simulink model "nonlinear_model"  (R2016a)
settings: Solver=VariableStepAuto  StartTime=0.0  StopTime=T  MaxStep=1e-3  RelTol=1e-3
values from neighbouring files (symbols this model uses):
  a = 0.025    [constants.m]
  A = [ 0     0     0     0     1     0     0     0 ... (first row only)    [reduced_state_space.m]
  angular_velocity_0 = [0 0 0]    [simulation.m]
  B = [0 0 0 0 b_11 0    0    b_51 ... (first row only)    [reduced_state_space.m]
  C = [c_11 0    0    c_15 0 0 0 0 ... (first row only)    [reduced_state_space.m]
  g = 9.81305    [constants.m]
  h = 0.0095    [constants.m]
  I = [I_1  0    0 ... (first row only)    [constants.m]
  K = lqr(A, B, Q, R)    [reduced_state_space.m]
  Kr = (lqr(A',C',Q_r,R_r))'    [reduced_state_space.m]
  Ks = pocet_zavitu * prumerna_area    (= 0.0603185789489)    [constants.m]
  m = pi*r^2*h*neodymium_density    (= 0.0694645405617)    [constants.m]
  m_0 = 3.3906    [constants.m]
  m_2 = 1.5321    [constants.m]
  max_I = 2    [constants.m]
  noise_power = 1*10^(-11)    (= 1e-11)    [constants.m]
  perm_vak_4pi = 10^(-7)    (= 1e-07)    [constants.m]
  phi_0 = [0.00 0.00 0]    [simulation.m]
  R = [1 0 ... (first row only)    [reduced_state_space.m]
  rot_damp = 0*0.00002    (= 0)    [constants.m]
  s = 1*0.001    (= 0.001)    [constants.m]
  sample_period = 0.003    [constants.m]
  setpoint_x = perm_vak_4pi*m_0 * ( (3*s*z_r)/(s^2+z_r^2)^(5/2) )    [simulation.m]
  setpoint_y = setpoint_x    [simulation.m]
  x_0 = [0.001 -0.0015 z_r-0.000]    [simulation.m]
  x_1 = [-a  a 0]    [constants.m]
  x_2 = [ a  a 0]    [constants.m]
  x_3 = [-a -a 0]    [constants.m]
  x_4 = [ a -a 0]    [constants.m]
  x_5 = [ 0  a 0]    [constants.m]
  x_6 = [-a  0 0]    [constants.m]
  x_7 = [ a  0 0]    [constants.m]
  x_8 = [ 0 -a 0]    [constants.m]
undefined symbols (not defined in the file or in its folder): Kd, Ki, Kp, X, Y, Z
libraries: sm_lib x27, nesl_utility x9, simulink x8, vrlib x1
(part 2 of 2)

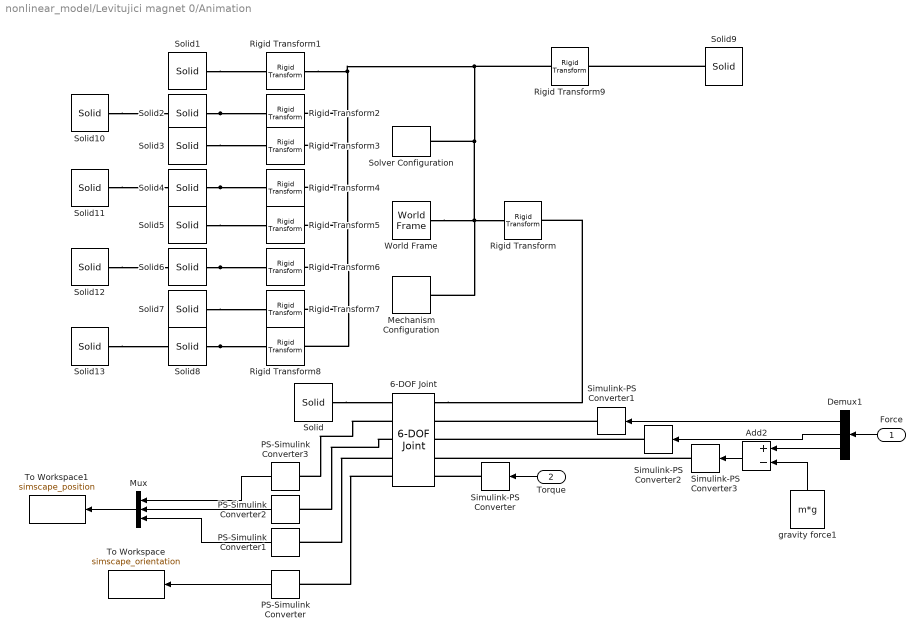
== system nonlinear_model/Levitujici magnet 0/Animation ==
  Force : Inport
  Torque : Inport  Port=2
  6-DOF Joint : sm_lib/Joints/6-DOF Joint  SenseConstraintForce=off  SenseConstraintForceX=off  SenseConstraintForceY=off  SenseConstraintForceZ=off  SenseConstraintTorque=off  SenseConstraintTorqueX=off  SenseConstraintTorqueY=off  SenseConstraintTorqueZ=off  SenseTotalForce=off  SenseTotalForceX=off  SenseTotalForceY=off  SenseTotalForceZ=off  SenseTotalTorque=off  SenseTotalTorqueX=off  SenseTotalTorqueY=off  SenseTotalTorqueZ=off  CompositeWrenchDir=FollowerOnBase  CompositeWrenchFrame=BaseFrame  PxEquilibriumPosition=0  PxEquilibriumPositionUnits=m  PxSpringStiffness=0  PxSpringStiffnessUnits=N/m  PxDampingCoefficient=0  PxDampingCoefficientUnits=N/(m/s)  PxTorqueActuationMode=InputTorque  PxMotionActuationMode=ComputedMotion  PxSensePosition=on  PxSenseVelocity=off  PxSenseAcceleration=off  PxSenseTorqueForce=off  PxPositionTargetSpecify=on  PxPositionTargetPriority=High  PxPositionTargetValue=x_0(1)  PxPositionTargetValueUnits=m  PxVelocityTargetSpecify=off  PxVelocityTargetPriority=High  PxVelocityTargetValue=0  PxVelocityTargetValueUnits=m/s  PyEquilibriumPosition=0  PyEquilibriumPositionUnits=m  PySpringStiffness=0  PySpringStiffnessUnits=N/m  PyDampingCoefficient=0  PyDampingCoefficientUnits=N/(m/s)  PyTorqueActuationMode=InputTorque  PyMotionActuationMode=ComputedMotion  PySensePosition=on  PySenseVelocity=off  PySenseAcceleration=off  PySenseTorqueForce=off  PyPositionTargetSpecify=on  PyPositionTargetPriority=High  PyPositionTargetValue=x_0(2)  PyPositionTargetValueUnits=m  PyVelocityTargetSpecify=off  PyVelocityTargetPriority=High  PyVelocityTargetValue=0  PyVelocityTargetValueUnits=m/s  PzEquilibriumPosition=0  PzEquilibriumPositionUnits=m  PzSpringStiffness=0  PzSpringStiffnessUnits=N/m  PzDampingCoefficient=0  PzDampingCoefficientUnits=N/(m/s)  PzTorqueActuationMode=InputTorque  PzMotionActuationMode=ComputedMotion  PzSensePosition=on  PzSenseVelocity=off  PzSenseAcceleration=off  PzSenseTorqueForce=off  PzPositionTargetSpecify=on  PzPositionTargetPriority=High  PzPositionTargetValue=x_0(3)  PzPositionTargetValueUnits=m  PzVelocityTargetSpecify=off  PzVelocityTargetPriority=High  PzVelocityTargetValue=0  PzVelocityTargetValueUnits=m/s  SphDefPosRotationMethod=None  SphDefPosRotationAngleUnits=deg  SphDefPosRotationStandardAxis=+Z  SphDefPosRotationAngle=0.0  SphDefPosRotationArbitraryAxis=[0 0 1]  SphDefPosFollAlignAxisA=+X  SphDefPosBaseAlignAxisA=+Y  SphDefPosFollAlignAxisB=+Y  SphDefPosBaseAlignAxisB=+Z  SphDefPosRotationSequenceAxes=FollowerAxes  SphDefPosRotationSequence=XYX  SphDefPosRotationSequenceAngles=[0 0 0]  SphDefPosRotationSequenceAnglesUnits=deg  SphDefPosRotationMatrix=[1 0 0; 0 1 0; 0 0 1]  SphEqPosRotationMethod=None  SphEqPosRotationAngleUnits=deg  SphEqPosRotationStandardAxis=+Z  SphEqPosRotationAngle=0.0  SphEqPosRotationArbitraryAxis=[0 0 1]  SphEqPosFollAlignAxisA=+X  SphEqPosBaseAlignAxisA=+Y  SphEqPosFollAlignAxisB=+Y  SphEqPosBaseAlignAxisB=+Z  SphEqPosRotationSequenceAxes=FollowerAxes  SphEqPosRotationSequence=XYX  SphEqPosRotationSequenceAngles=[0 0 0]  SphEqPosRotationSequenceAnglesUnits=deg  SphEqPosRotationMatrix=[1 0 0; 0 1 0; 0 0 1]  SphSpringStiffness=0  SphSpringStiffnessUnits=N*m/deg  SphDampingCoefficient=rot_damp_sim  SphDampingCoefficientUnits=N*m/(deg/s)  SphActuateTorqueX=off  SphActuateTorqueY=off  SphActuateTorqueZ=off  SphActuateTorque=on  SphTorqueActuationMode=InputTorque  SphMotionActuationMode=ComputedMotion  SphActuationFrame=BaseFrame  SphSensePosition=on  SphSenseVelocityX=off  SphSenseVelocityY=off  SphSenseVelocityZ=off  SphSenseVelocity=off  SphSenseAccelerationX=off  SphSenseAccelerationY=off  SphSenseAccelerationZ=off  SphSenseAcceleration=off  SphSenseTorqueX=off  SphSenseTorqueY=off  SphSenseTorqueZ=off  SphSenseTorqueForce=off  SphSensingFrame=BaseFrame  SphPositionTargetRotationMethod=RotationSequence  SphPositionTargetRotationAngleUnits=deg  SphPositionTargetRotationStandardAxis=+Z  SphPositionTargetRotationAngle=0.0  SphPositionTargetRotationArbitraryAxis=[0 0 1]  SphPositionTargetFollAlignAxisA=+X  SphPositionTargetBaseAlignAxisA=+Y  SphPositionTargetFollAlignAxisB=+Y  SphPositionTargetBaseAlignAxisB=+Z  SphPositionTargetRotationSequenceAxes=FollowerAxes  SphPositionTargetRotationSequence=ZYX  SphPositionTargetRotationSequenceAngles=[phi_0(3), phi_0(2), phi_0(1)]  SphPositionTargetRotationSequenceAnglesUnits=rad  SphPositionTargetRotationMatrix=[1 0 0; 0 1 0; 0 0 1]  SphPositionTargetSpecify=on  SphPositionTargetPriority=High  SphVelocityTargetValue=[angular_velocity_0(3), angular_velocity_0(2), angular_velocity_0(1)]  SphVelocityTargetValueUnits=deg/s  SphVelocityTargetSpecify=on  SphVelocityTargetPriority=High  SphVelocityTargetInFollowerFrame=on
  Add2 : Sum  Inputs=+-
  Demux1 : Demux  Outputs=3
  Mechanism Configuration : sm_lib/Utilities/Mechanism Configuration  UniformGravity=Constant  GravityVector=[0 0 -0]  GravityUnits=m/s^2  LinearizationDelta=0.001
  Mux : Mux  Inputs=3
  PS-Simulink Converter{,1..3} (4 alike) : nesl_utility/PS-Simulink Converter  PhysicalDomain=network_engine_domain  SubClassName=ps_output  LeftPortType=input  RightPortType=output  PseudoPeriodic=off  Frequencies=[]  Unit=1  AffineConversion=off
  Rigid Transform : sm_lib/Frames and Transforms/Rigid Transform  TranslationMethod=None  TranslationLengthUnit=m  TranslationStandardAxis=+Z  TranslationStandardOffset=0  TranslationCartesianOffset=[]  TranslationROffset=0  TranslationROffsetUnits=m  TranslationZOffset=0  TranslationZOffsetUnits=m  TranslationThetaOffset=0  TranslationThetaOffsetUnits=deg  RotationMethod=None  RotationAngleUnits=deg  RotationStandardAxis=+Z  RotationAngle=0.0  RotationArbitraryAxis=[0 0 1]  FollAlignAxisA=+X  BaseAlignAxisA=+Y  FollAlignAxisB=+Y  BaseAlignAxisB=+Z  RotationSequenceAxes=FollowerAxes  RotationSequence=ZXY  RotationSequenceAngles=[phi_0(3), phi_0(2), phi_0(1)]  RotationSequenceAnglesUnits=rad  RotationMatrix=[1 0 0; 0 1 0; 0 0 1]
  Rigid Transform1 : sm_lib/Frames and Transforms/Rigid Transform  TranslationMethod=Cartesian  TranslationLengthUnit=m  TranslationStandardAxis=+Z  TranslationStandardOffset=0  TranslationCartesianOffset=x_1-[0 0 0.0055]  TranslationROffset=0  TranslationROffsetUnits=m  TranslationZOffset=0  TranslationZOffsetUnits=m  TranslationThetaOffset=0  TranslationThetaOffsetUnits=deg  RotationMethod=None  RotationAngleUnits=deg  RotationStandardAxis=+Z  RotationAngle=0.0  RotationArbitraryAxis=[0 0 1]  FollAlignAxisA=+X  BaseAlignAxisA=+Y  FollAlignAxisB=+Y  BaseAlignAxisB=+Z  RotationSequenceAxes=FollowerAxes  RotationSequence=XYX  RotationSequenceAngles=[0 0 0]  RotationSequenceAnglesUnits=deg  RotationMatrix=[1 0 0; 0 1 0; 0 0 1]
  Rigid Transform2 : sm_lib/Frames and Transforms/Rigid Transform  TranslationMethod=Cartesian  TranslationLengthUnit=m  TranslationStandardAxis=+Z  TranslationStandardOffset=0  TranslationCartesianOffset=x_5-[0 0 0.0055]  TranslationROffset=0  TranslationROffsetUnits=m  TranslationZOffset=0  TranslationZOffsetUnits=m  TranslationThetaOffset=0  TranslationThetaOffsetUnits=deg  RotationMethod=None  RotationAngleUnits=deg  RotationStandardAxis=+Z  RotationAngle=0.0  RotationArbitraryAxis=[0 0 1]  FollAlignAxisA=+X  BaseAlignAxisA=+Y  FollAlignAxisB=+Y  BaseAlignAxisB=+Z  RotationSequenceAxes=FollowerAxes  RotationSequence=XYX  RotationSequenceAngles=[0 0 0]  RotationSequenceAnglesUnits=deg  RotationMatrix=[1 0 0; 0 1 0; 0 0 1]
  Rigid Transform3 : sm_lib/Frames and Transforms/Rigid Transform  TranslationMethod=Cartesian  TranslationLengthUnit=m  TranslationStandardAxis=+Z  TranslationStandardOffset=0  TranslationCartesianOffset=x_2-[0 0 0.0055]  TranslationROffset=0  TranslationROffsetUnits=m  TranslationZOffset=0  TranslationZOffsetUnits=m  TranslationThetaOffset=0  TranslationThetaOffsetUnits=deg  RotationMethod=None  RotationAngleUnits=deg  RotationStandardAxis=+Z  RotationAngle=0.0  RotationArbitraryAxis=[0 0 1]  FollAlignAxisA=+X  BaseAlignAxisA=+Y  FollAlignAxisB=+Y  BaseAlignAxisB=+Z  RotationSequenceAxes=FollowerAxes  RotationSequence=XYX  RotationSequenceAngles=[0 0 0]  RotationSequenceAnglesUnits=deg  RotationMatrix=[1 0 0; 0 1 0; 0 0 1]
  Rigid Transform4 : sm_lib/Frames and Transforms/Rigid Transform  TranslationMethod=Cartesian  TranslationLengthUnit=m  TranslationStandardAxis=+Z  TranslationStandardOffset=0  TranslationCartesianOffset=x_6-[0 0 0.0055]  TranslationROffset=0  TranslationROffsetUnits=m  TranslationZOffset=0  TranslationZOffsetUnits=m  TranslationThetaOffset=0  TranslationThetaOffsetUnits=deg  RotationMethod=None  RotationAngleUnits=deg  RotationStandardAxis=+Z  RotationAngle=0.0  RotationArbitraryAxis=[0 0 1]  FollAlignAxisA=+X  BaseAlignAxisA=+Y  FollAlignAxisB=+Y  BaseAlignAxisB=+Z  RotationSequenceAxes=FollowerAxes  RotationSequence=XYX  RotationSequenceAngles=[0 0 0]  RotationSequenceAnglesUnits=deg  RotationMatrix=[1 0 0; 0 1 0; 0 0 1]
  Rigid Transform5 : sm_lib/Frames and Transforms/Rigid Transform  TranslationMethod=Cartesian  TranslationLengthUnit=m  TranslationStandardAxis=+Z  TranslationStandardOffset=0  TranslationCartesianOffset=x_3-[0 0 0.0055]  TranslationROffset=0  TranslationROffsetUnits=m  TranslationZOffset=0  TranslationZOffsetUnits=m  TranslationThetaOffset=0  TranslationThetaOffsetUnits=deg  RotationMethod=None  RotationAngleUnits=deg  RotationStandardAxis=+Z  RotationAngle=0.0  RotationArbitraryAxis=[0 0 1]  FollAlignAxisA=+X  BaseAlignAxisA=+Y  FollAlignAxisB=+Y  BaseAlignAxisB=+Z  RotationSequenceAxes=FollowerAxes  RotationSequence=XYX  RotationSequenceAngles=[0 0 0]  RotationSequenceAnglesUnits=deg  RotationMatrix=[1 0 0; 0 1 0; 0 0 1]
  Rigid Transform6 : sm_lib/Frames and Transforms/Rigid Transform  TranslationMethod=Cartesian  TranslationLengthUnit=m  TranslationStandardAxis=+Z  TranslationStandardOffset=0  TranslationCartesianOffset=x_7-[0 0 0.0055]  TranslationROffset=0  TranslationROffsetUnits=m  TranslationZOffset=0  TranslationZOffsetUnits=m  TranslationThetaOffset=0  TranslationThetaOffsetUnits=deg  RotationMethod=None  RotationAngleUnits=deg  RotationStandardAxis=+Z  RotationAngle=0.0  RotationArbitraryAxis=[0 0 1]  FollAlignAxisA=+X  BaseAlignAxisA=+Y  FollAlignAxisB=+Y  BaseAlignAxisB=+Z  RotationSequenceAxes=FollowerAxes  RotationSequence=XYX  RotationSequenceAngles=[0 0 0]  RotationSequenceAnglesUnits=deg  RotationMatrix=[1 0 0; 0 1 0; 0 0 1]
  Rigid Transform7 : sm_lib/Frames and Transforms/Rigid Transform  TranslationMethod=Cartesian  TranslationLengthUnit=m  TranslationStandardAxis=+Z  TranslationStandardOffset=0  TranslationCartesianOffset=x_4-[0 0 0.0055]  TranslationROffset=0  TranslationROffsetUnits=m  TranslationZOffset=0  TranslationZOffsetUnits=m  TranslationThetaOffset=0  TranslationThetaOffsetUnits=deg  RotationMethod=None  RotationAngleUnits=deg  RotationStandardAxis=+Z  RotationAngle=0.0  RotationArbitraryAxis=[0 0 1]  FollAlignAxisA=+X  BaseAlignAxisA=+Y  FollAlignAxisB=+Y  BaseAlignAxisB=+Z  RotationSequenceAxes=FollowerAxes  RotationSequence=XYX  RotationSequenceAngles=[0 0 0]  RotationSequenceAnglesUnits=deg  RotationMatrix=[1 0 0; 0 1 0; 0 0 1]
  Rigid Transform8 : sm_lib/Frames and Transforms/Rigid Transform  TranslationMethod=Cartesian  TranslationLengthUnit=m  TranslationStandardAxis=+Z  TranslationStandardOffset=0  TranslationCartesianOffset=x_8-[0 0 0.0055]  TranslationROffset=0  TranslationROffsetUnits=m  TranslationZOffset=0  TranslationZOffsetUnits=m  TranslationThetaOffset=0  TranslationThetaOffsetUnits=deg  RotationMethod=None  RotationAngleUnits=deg  RotationStandardAxis=+Z  RotationAngle=0.0  RotationArbitraryAxis=[0 0 1]  FollAlignAxisA=+X  BaseAlignAxisA=+Y  FollAlignAxisB=+Y  BaseAlignAxisB=+Z  RotationSequenceAxes=FollowerAxes  RotationSequence=XYX  RotationSequenceAngles=[0 0 0]  RotationSequenceAnglesUnits=deg  RotationMatrix=[1 0 0; 0 1 0; 0 0 1]
  Rigid Transform9 : sm_lib/Frames and Transforms/Rigid Transform  TranslationMethod=Cartesian  TranslationLengthUnit=m  TranslationStandardAxis=+Z  TranslationStandardOffset=0  TranslationCartesianOffset=[0 0 -0.0165]  TranslationROffset=0  TranslationROffsetUnits=m  TranslationZOffset=0  TranslationZOffsetUnits=m  TranslationThetaOffset=0  TranslationThetaOffsetUnits=deg  RotationMethod=None  RotationAngleUnits=deg  RotationStandardAxis=+Z  RotationAngle=0.0  RotationArbitraryAxis=[0 0 1]  FollAlignAxisA=+X  BaseAlignAxisA=+Y  FollAlignAxisB=+Y  BaseAlignAxisB=+Z  RotationSequenceAxes=FollowerAxes  RotationSequence=XYX  RotationSequenceAngles=[0 0 0]  RotationSequenceAnglesUnits=deg  RotationMatrix=[1 0 0; 0 1 0; 0 0 1]
  Simulink-PS Converter{,1..3} (4 alike) : nesl_utility/Simulink-PS Converter  PhysicalDomain=network_engine_domain  SubClassName=ps_input  LeftPortType=input  RightPortType=output  PseudoPeriodic=off  Frequencies=[]  NoiseDistribution=none  NoiseParameters=[]  Unit=1  AffineConversion=off  InputFiltering=off  SimscapeFilterOrder=1  InputFilterTimeConstant=0.001  UdotUserProvided=1
  Solid : sm_lib/Body Elements/Solid  InertiaType=CalculateFromGeometry  Mass=m  MassUnits=kg  CenterOfMass=[0 0 0]  CenterOfMassUnits=m  MomentsOfInertia=[1 1 1]  MomentsOfInertiaUnits=kg*m^2  ProductsOfInertia=[0 0 0]  ProductsOfInertiaUnits=kg*m^2  DensityBased=off  Density=neodymium_density  DensityUnits=kg/(m^3)  DoExposeReferenceFrame=on  SerializedFrames=<Frames/>  GraphicType=FromGeometry  MarkerShape=Sphere  MarkerSize=10  GraphicVisPropType=SimpleVisualProperties  GraphicDiffuseColor=[0.5 0.5 0.5]  GraphicSpecularColor=[0.5 0.5 0.5 1.0]  GraphicAmbientColor=[0.15 0.15 0.15 1.0]  GraphicEmissiveColor=[0.0 0.0 0.0 1.0]  GraphicShininess=75  GraphicOpacity=1.0  GeometryShape=Cylinder  RectangleSize=[1 1]  RectangleSizeUnits=m  BrickDimensions=[1 1 1]  BrickDimensionUnits=m  CylinderRadius=r  CylinderRadiusUnits=m  CylinderLength=h  CylinderLengthUnits=m  SphereRadius=1  SphereRadiusUnits=m  EllipsoidRadii=[1 1 1]  EllipsoidRadiiUnits=m  ExtrusionCrossSection=[1 1; -1 1; -1 -1; 1 -1]  ExtrusionCrossSectionUnits=m  ExtrusionLength=1  ExtrusionLengthUnits=m  PolygonNumSides=3  PolygonOuterRadius=1  PolygonOuterRadiusUnits=m  ExtGeomFileType=STEP  ExtGeomFileUnits=m  RevolutionCrossSection=[1 1; 1 -1; 2 -1; 2 1]  RevolutionCrossSectionUnits=m  RevolutionExtent=Full  RevolutionAngle=180  RevolutionAngleUnits=deg
  Solid{1,3,5,7} (4 alike) : sm_lib/Body Elements/Solid  InertiaType=CalculateFromGeometry  Mass=m  MassUnits=kg  CenterOfMass=[0 0 0]  CenterOfMassUnits=m  MomentsOfInertia=[1 1 1]  MomentsOfInertiaUnits=kg*m^2  ProductsOfInertia=[0 0 0]  ProductsOfInertiaUnits=kg*m^2  DensityBased=off  Density=1000  DensityUnits=kg/(m^3)  DoExposeReferenceFrame=on  SerializedFrames=<Frames/>  GraphicType=FromGeometry  MarkerShape=Sphere  MarkerSize=10  GraphicVisPropType=SimpleVisualProperties  GraphicDiffuseColor=[0.5 0.5 0.5]  GraphicSpecularColor=[0.5 0.5 0.5 1.0]  GraphicAmbientColor=[0.15 0.15 0.15 1.0]  GraphicEmissiveColor=[0.0 0.0 0.0 1.0]  GraphicShininess=75  GraphicOpacity=1.0  GeometryShape=Cylinder  RectangleSize=[1 1]  RectangleSizeUnits=m  BrickDimensions=[1 1 1]  BrickDimensionUnits=m  CylinderRadius=0.0075  CylinderRadiusUnits=m  CylinderLength=0.011  CylinderLengthUnits=m  SphereRadius=1  SphereRadiusUnits=m  EllipsoidRadii=[1 1 1]  EllipsoidRadiiUnits=m  ExtrusionCrossSection=[1 1; -1 1; -1 -1; 1 -1]  ExtrusionCrossSectionUnits=m  ExtrusionLength=1  ExtrusionLengthUnits=m  PolygonNumSides=3  PolygonOuterRadius=1  PolygonOuterRadiusUnits=m  ExtGeomFileType=STEP  ExtGeomFileUnits=m  RevolutionCrossSection=[1 1; 1 -1; 2 -1; 2 1]  RevolutionCrossSectionUnits=m  RevolutionExtent=Full  RevolutionAngle=180  RevolutionAngleUnits=deg
  Solid{10..13} (4 alike) : sm_lib/Body Elements/Solid  InertiaType=CalculateFromGeometry  Mass=m  MassUnits=kg  CenterOfMass=[0 0 0]  CenterOfMassUnits=m  MomentsOfInertia=[1 1 1]  MomentsOfInertiaUnits=kg*m^2  ProductsOfInertia=[0 0 0]  ProductsOfInertiaUnits=kg*m^2  DensityBased=off  Density=1000  DensityUnits=kg/(m^3)  DoExposeReferenceFrame=on  SerializedFrames=<Frames/>  GraphicType=FromGeometry  MarkerShape=Sphere  MarkerSize=10  GraphicVisPropType=SimpleVisualProperties  GraphicDiffuseColor=[0.8 0.8 0.8]  GraphicSpecularColor=[0.5 0.5 0.5 1.0]  GraphicAmbientColor=[0.15 0.15 0.15 1.0]  GraphicEmissiveColor=[0.0 0.0 0.0 1.0]  GraphicShininess=75  GraphicOpacity=1.0  GeometryShape=Cylinder  RectangleSize=[1 1]  RectangleSizeUnits=m  BrickDimensions=[1 1 1]  BrickDimensionUnits=m  CylinderRadius=0.004  CylinderRadiusUnits=m  CylinderLength=0.0111  CylinderLengthUnits=m  SphereRadius=1  SphereRadiusUnits=m  EllipsoidRadii=[1 1 1]  EllipsoidRadiiUnits=m  ExtrusionCrossSection=[1 1; -1 1; -1 -1; 1 -1]  ExtrusionCrossSectionUnits=m  ExtrusionLength=1  ExtrusionLengthUnits=m  PolygonNumSides=3  PolygonOuterRadius=1  PolygonOuterRadiusUnits=m  ExtGeomFileType=STEP  ExtGeomFileUnits=m  RevolutionCrossSection=[1 1; 1 -1; 2 -1; 2 1]  RevolutionCrossSectionUnits=m  RevolutionExtent=Full  RevolutionAngle=180  RevolutionAngleUnits=deg
  Solid{2,4,6,8} (4 alike) : sm_lib/Body Elements/Solid  InertiaType=CalculateFromGeometry  Mass=m  MassUnits=kg  CenterOfMass=[0 0 0]  CenterOfMassUnits=m  MomentsOfInertia=[1 1 1]  MomentsOfInertiaUnits=kg*m^2  ProductsOfInertia=[0 0 0]  ProductsOfInertiaUnits=kg*m^2  DensityBased=off  Density=1000  DensityUnits=kg/(m^3)  DoExposeReferenceFrame=on  SerializedFrames=<Frames/>  GraphicType=FromGeometry  MarkerShape=Sphere  MarkerSize=10  GraphicVisPropType=SimpleVisualProperties  GraphicDiffuseColor=[1.0 0.6 0.2]  GraphicSpecularColor=[0.5 0.5 0.5 1.0]  GraphicAmbientColor=[0.15 0.15 0.15 1.0]  GraphicEmissiveColor=[0.0 0.0 0.0 1.0]  GraphicShininess=75  GraphicOpacity=1.0  GeometryShape=Cylinder  RectangleSize=[1 1]  RectangleSizeUnits=m  BrickDimensions=[1 1 1]  BrickDimensionUnits=m  CylinderRadius=0.009  CylinderRadiusUnits=m  CylinderLength=0.011  CylinderLengthUnits=m  SphereRadius=1  SphereRadiusUnits=m  EllipsoidRadii=[1 1 1]  EllipsoidRadiiUnits=m  ExtrusionCrossSection=[1 1; -1 1; -1 -1; 1 -1]  ExtrusionCrossSectionUnits=m  ExtrusionLength=1  ExtrusionLengthUnits=m  PolygonNumSides=3  PolygonOuterRadius=1  PolygonOuterRadiusUnits=m  ExtGeomFileType=STEP  ExtGeomFileUnits=m  RevolutionCrossSection=[1 1; 1 -1; 2 -1; 2 1]  RevolutionCrossSectionUnits=m  RevolutionExtent=Full  RevolutionAngle=180  RevolutionAngleUnits=deg
  Solid9 : sm_lib/Body Elements/Solid  InertiaType=CalculateFromGeometry  Mass=m  MassUnits=kg  CenterOfMass=[0 0 0]  CenterOfMassUnits=m  MomentsOfInertia=[1 1 1]  MomentsOfInertiaUnits=kg*m^2  ProductsOfInertia=[0 0 0]  ProductsOfInertiaUnits=kg*m^2  DensityBased=off  Density=1000  DensityUnits=kg/(m^3)  DoExposeReferenceFrame=on  SerializedFrames=<Frames/>  GraphicType=FromGeometry  MarkerShape=Sphere  MarkerSize=10  GraphicVisPropType=SimpleVisualProperties  GraphicDiffuseColor=[0.6 0.2 0.0]  GraphicSpecularColor=[0.5 0.5 0.5 1.0]  GraphicAmbientColor=[0.15 0.15 0.15 1.0]  GraphicEmissiveColor=[0.0 0.0 0.0 1.0]  GraphicShininess=75  GraphicOpacity=1.0  GeometryShape=Brick  RectangleSize=[1 1]  RectangleSizeUnits=m  BrickDimensions=[2*a+0.02 2*a+0.02 0.011]  BrickDimensionUnits=m  CylinderRadius=R/3  CylinderRadiusUnits=m  CylinderLength=h*3  CylinderLengthUnits=m  SphereRadius=a  SphereRadiusUnits=m  EllipsoidRadii=[1 1 1]  EllipsoidRadiiUnits=m  ExtrusionCrossSection=[1 1; -1 1; -1 -1; 1 -1]  ExtrusionCrossSectionUnits=m  ExtrusionLength=1  ExtrusionLengthUnits=m  PolygonNumSides=3  PolygonOuterRadius=1  PolygonOuterRadiusUnits=m  ExtGeomFileType=STEP  ExtGeomFileUnits=m  RevolutionCrossSection=[1 1; 1 -1; 2 -1; 2 1]  RevolutionCrossSectionUnits=m  RevolutionExtent=Full  RevolutionAngle=180  RevolutionAngleUnits=deg
  Solver Configuration : nesl_utility/Solver Configuration  PhysicalDomain=network_engine_domain  SubClassName=solver  LeftPortType=input  RightPortType=generic  Accelerate=off  Tones=[]  Harmonics=[]  SimulateNoise=off  Profile=off  UseLocalSampling=off  EnableSwitchedLinearOptims=on  FrequencyDomain=off  UseCCode=off  RelTol=0.001  AbsTol=1e-06  MinStep=1e-09  ToWorkspace=off  RevertToSquareIcSolve=off  NumHomotopyIterations=100  PhasorMode=off  PhasorModeNumHarmonics=1  OverrideAbsTol=off  DoDC=off  ResidualTolerance=1e-09  UseLocalSolver=off  LocalSolverChoice=NE_BACKWARD_EULER_ADVANCER  LocalSolverSampleTime=0.001  DoFixedCost=off  MaxNonlinIter=3  MaxModeIter=2  LinearAlgebra=Sparse  DelaysMemoryBudget=1024  AutomaticFiltering=on  FilteringTimeConstant=0.001
  To Workspace : ToWorkspace  VariableName=simscape_orientation  SaveFormat=Timeseries  SampleTime=-1
  To Workspace1 : ToWorkspace  VariableName=simscape_position  SaveFormat=Timeseries  SampleTime=-1
  World Frame : sm_lib/Frames and Transforms/World Frame
  gravity force1 : Constant  Value=m*g
  wires:
  Demux1/3 -> Add2/1
  Force/1 -> Demux1/1
  gravity force1/1 -> Add2/2
  Torque/1 -> Simulink-PS Converter/1
  Demux1/1 -> Simulink-PS Converter1/1
  Demux1/2 -> Simulink-PS Converter2/1
  Add2/1 -> Simulink-PS Converter3/1
  PS-Simulink Converter/1 -> To Workspace/1
  PS-Simulink Converter3/1 -> Mux/1
  PS-Simulink Converter2/1 -> Mux/2
  Mux/1 -> To Workspace1/1
  PS-Simulink Converter1/1 -> Mux/3
  connections:
  Simulink-PS Converter1/RConn1 -- 6-DOF Joint/LConn2
  Simulink-PS Converter2/RConn1 -- 6-DOF Joint/LConn3
  Simulink-PS Converter/RConn1 -- 6-DOF Joint/LConn5
  Solid/RConn1 -- 6-DOF Joint/RConn1
  Mechanism Configuration/RConn1 -- Rigid Transform/LConn1 -- World Frame/RConn1 -- Rigid Transform2/LConn1 -- Rigid Transform3/LConn1 -- Rigid Transform4/LConn1 -- Rigid Transform5/LConn1 -- Rigid Transform6/LConn1 -- Rigid Transform7/LConn1 -- Rigid Transform8/LConn1 -- Rigid Transform1/LConn1 -- Rigid Transform9/LConn1 -- Solver Configuration/RConn1
  Solid9/RConn1 -- Rigid Transform9/RConn1
  Simulink-PS Converter3/RConn1 -- 6-DOF Joint/LConn4
  Solid1/RConn1 -- Rigid Transform1/RConn1
  Solid2/RConn1 -- Rigid Transform2/RConn1 -- Solid10/RConn1
  Solid3/RConn1 -- Rigid Transform3/RConn1
  Solid4/RConn1 -- Rigid Transform4/RConn1 -- Solid11/RConn1
  Solid5/RConn1 -- Rigid Transform5/RConn1
  Solid6/RConn1 -- Rigid Transform6/RConn1 -- Solid12/RConn1
  Solid7/RConn1 -- Rigid Transform7/RConn1
  Solid8/RConn1 -- Rigid Transform8/RConn1 -- Solid13/RConn1
  6-DOF Joint/LConn1 -- Rigid Transform/RConn1
  6-DOF Joint/RConn5 -- PS-Simulink Converter/LConn1
  6-DOF Joint/RConn2 -- PS-Simulink Converter3/LConn1
  6-DOF Joint/RConn3 -- PS-Simulink Converter2/LConn1
  6-DOF Joint/RConn4 -- PS-Simulink Converter1/LConn1

== system nonlinear_model/Levitujici magnet 0/Orientation computation ==
  note: torque
  note: Inertia matrix
  In1 : Inport
  " " : Gain  Gain=I  Multiplication=Matrix(K*u)
  1/Inertia matrix : Gain  Gain=eye(3)/I  Multiplication=Matrix(K*u)
  Add1 : Sum  Inputs=+--
  Angular velocity to Euler angles rates : Subsystem
  Cross Product : vrlib/Utilities/Cross Product
  Gain : Gain  Gain=rot_damp
  Integrator2 : Integrator  InitialCondition=angular_velocity_0
  Integrator3 : Integrator  InitialCondition=phi_0
  World frame to Body frame : Subsystem
  Out1 : Outport
  wires:
  Integrator2/1 -> Angular velocity to Euler angles rates/1(Angular velocity), " "/1, Cross Product/2, Gain/1  "angular velocity"
  Integrator3/1 -> Out1/1, World frame to Body frame/1(World frame Euler angles), Angular velocity to Euler angles rates/2(Euler angles)  "euler angles"
  Add1/1 -> 1/Inertia matrix/1
  " "/1 -> Cross Product/1
  Cross Product/1 -> Add1/2  "gyroscopic torque"
  World frame to Body frame/1(Body frame Vector) -> Add1/1
  Angular velocity to Euler angles rates/1(Euler angles rates) -> Integrator3/1
  Gain/1 -> Add1/3
  1/Inertia matrix/1 -> Integrator2/1
  In1/1 -> World frame to Body frame/2(World frame Vector)

== system nonlinear_model/Levitujici magnet 0/Position computation ==
  Force : Inport
  1/mass : Gain  Gain=1/m
  Add : Sum  Inputs=+-
  Demux : Demux  Outputs=3
  Integrator : Integrator
  Integrator1 : Integrator  InitialCondition=x_0
  Mux : Mux  Inputs=3
  gravity force : Constant  Value=m*g
  Position : Outport
  wires:
  Integrator1/1 -> Position/1  "[x, y, z]"
  Add/1 -> Mux/3
  Force/1 -> Demux/1
  Demux/3 -> Add/1
  gravity force/1 -> Add/2
  Integrator/1 -> Integrator1/1
  Demux/2 -> Mux/2
  Mux/1 -> 1/mass/1
  Demux/1 -> Mux/1
  1/mass/1 -> Integrator/1

== system nonlinear_model/Regulators/LQR with direct state measurement ==
  Position : Inport
  Orientation : Inport  Port=2
  Demux : Demux  Outputs=2
  Discrete Derivative : simulink/Discrete/Discrete Derivative  gainval=1.0  ICPrevScaledInput=0.0  OutMin=[]  OutMax=[]  OutDataType=fixdt(1, 16)  OutScaling=2^-10  DoSatur=off
  Gain : Gain  Gain=-K  Multiplication=Matrix(K*u)
  Mux : Mux  Inputs=2
  Mux1 : Mux  Inputs=2
  Saturation : Saturate  UpperLimit=max_I  LowerLimit=-max_I
  State selector : Gain  Gain=[1 0 0; 0 1 0]  Multiplication=Matrix(K*u)
  State selector1 : Gain  Gain=[1 0 0; 0 1 0]  Multiplication=Matrix(K*u)
  Zero-Order Hold : ZeroOrderHold  SampleTime=sample_period
  u_x : Outport
  u_y : Outport  Port=2
  wires:
  Demux/1 -> u_x/1
  Demux/2 -> u_y/1
  Mux/1 -> Gain/1
  Discrete Derivative/1 -> Mux/2
  Gain/1 -> Saturation/1
  Saturation/1 -> Demux/1
  Position/1 -> State selector/1
  Orientation/1 -> State selector1/1
  Mux1/1 -> Zero-Order Hold/1
  State selector/1 -> Mux1/1
  State selector1/1 -> Mux1/2
  Zero-Order Hold/1 -> Discrete Derivative/1, Mux/1

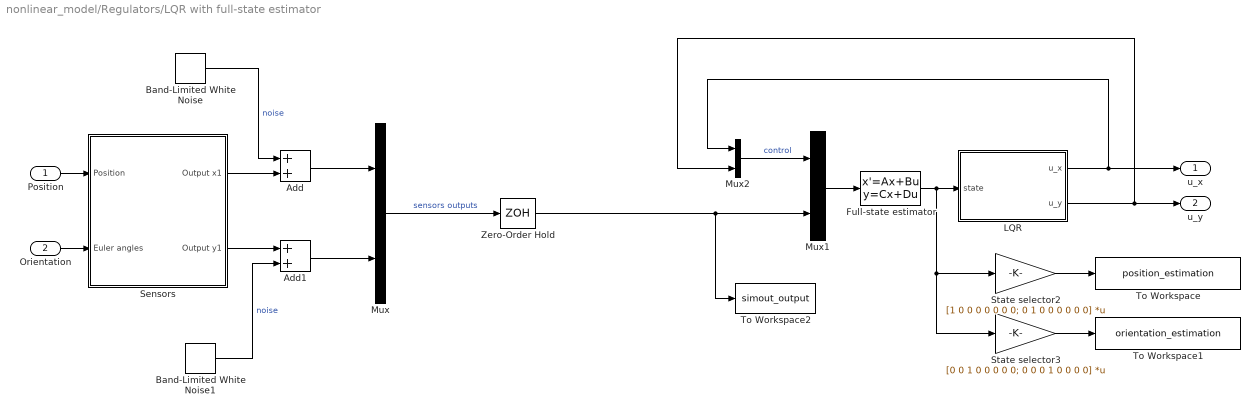
== system nonlinear_model/Regulators/LQR with full-state estimator ==
  Position : Inport
  Orientation : Inport  Port=2
  Add : Sum
  Add1 : Sum
  Band-Limited White Noise : simulink/Sources/Band-Limited White Noise  Cov=[noise_power]  Ts=sample_period  seed=[round(100000*rand)]
  Band-Limited White Noise1 : simulink/Sources/Band-Limited White Noise  Cov=[noise_power]  Ts=sample_period  seed=[round(100000*rand)]
  Full-state estimator : StateSpace  A=A-Kr*C  B=[B Kr]  C=eye(8)  D=0*[B Kr]  X0=0
  LQR : Subsystem
  Mux : Mux  Inputs=2
  Mux1 : Mux  Inputs=2
  Mux2 : Mux  Inputs=2
  Sensors : Subsystem
      mask Display: image(imread('obrazky/sensor.jpg'))
  State selector2 : Gain  Gain=[1 0 0 0 0 0 0 0; 0 1 0 0 0 0 0 0]  Multiplication=Matrix(K*u)
  State selector3 : Gain  Gain=[0 0 1 0 0 0 0 0; 0 0 0 1 0 0 0 0]  Multiplication=Matrix(K*u)
  To Workspace : ToWorkspace  VariableName=position_estimation  SaveFormat=Timeseries  SampleTime=-1
  To Workspace1 : ToWorkspace  VariableName=orientation_estimation  SaveFormat=Timeseries  SampleTime=-1
  To Workspace2 : ToWorkspace  VariableName=simout_output  SaveFormat=Timeseries  SampleTime=-1
  Zero-Order Hold : ZeroOrderHold  SampleTime=sample_period
  u_x : Outport
  u_y : Outport  Port=2
  wires:
  Mux1/1 -> Full-state estimator/1
  Full-state estimator/1 -> State selector2/1, State selector3/1, LQR/1(state)
  Mux2/1 -> Mux1/1  "control"
  LQR/1(u_x) -> Mux2/1, u_x/1
  LQR/2(u_y) -> u_y/1, Mux2/2
  Mux/1 -> Zero-Order Hold/1  "sensors outputs"
  State selector2/1 -> To Workspace/1
  State selector3/1 -> To Workspace1/1
  Position/1 -> Sensors/1(Position)
  Orientation/1 -> Sensors/2(Euler angles)
  Sensors/1(Output x1) -> Add/2
  Add/1 -> Mux/1
  Sensors/2(Output y1) -> Add1/1
  Add1/1 -> Mux/2
  Band-Limited White Noise1/1 -> Add1/2  "noise"
  Band-Limited White Noise/1 -> Add/1  "noise"
  Zero-Order Hold/1 -> To Workspace2/1, Mux1/2

== system nonlinear_model/Regulators/PID ==
  Position : Inport
  Orientation : Inport  Port=2
  Add : Sum
  Add1 : Sum
  Band-Limited White Noise : simulink/Sources/Band-Limited White Noise  Cov=[noise_power]  Ts=sample_period  seed=[round(100000*rand)]
  Band-Limited White Noise1 : simulink/Sources/Band-Limited White Noise  Cov=[noise_power]  Ts=sample_period  seed=[round(100000*rand)]
  Demux : Demux  Outputs=2
  Mux : Mux  Inputs=2
  PID X : Subsystem
  PID Y : Subsystem
  Sensors : Subsystem
      mask Display: image(imread('obrazky/sensor.jpg'))
  To Workspace2 : ToWorkspace  VariableName=simout_output  SaveFormat=Timeseries  SampleTime=-1
  Zero-Order Hold : ZeroOrderHold  SampleTime=sample_period
  u_x : Outport
  u_y : Outport  Port=2
  wires:
  Mux/1 -> Zero-Order Hold/1  "sensors outputs"
  Position/1 -> Sensors/1(Position)
  Orientation/1 -> Sensors/2(Euler angles)
  Sensors/1(Output x1) -> Add/2
  Add/1 -> Mux/1
  Sensors/2(Output y1) -> Add1/1
  Add1/1 -> Mux/2
  Band-Limited White Noise1/1 -> Add1/2  "noise"
  Band-Limited White Noise/1 -> Add/1  "noise"
  Zero-Order Hold/1 -> To Workspace2/1, Demux/1
  Demux/1 -> PID X/1(In1)
  Demux/2 -> PID Y/1(In1)
  PID X/1(Out1) -> u_x/1
  PID Y/1(Out1) -> u_y/1

== system nonlinear_model/Stable magnet 2/stop simulation ==
  "Relative position " : Inport
  Constant1 : Constant  Value=0
  Constant2 : Constant
  Stop Simulation : Stop
  Switch : Switch  Criteria=u2 > Threshold  Threshold=0.001
  norm : Fcn  Expr=sqrt(u(1)^2+u(2)^2+u(3)^2)
  wires:
  norm/1 -> Switch/2  "distance"
  Switch/1 -> Stop Simulation/1
  Constant1/1 -> Switch/1
  Constant2/1 -> Switch/3
  "Relative position "/1 -> norm/1

== system nonlinear_model/Stable magnet 4/stop simulation ==
  "Relative position " : Inport
  Constant1 : Constant  Value=0
  Constant2 : Constant
  Stop Simulation : Stop
  Switch : Switch  Criteria=u2 > Threshold  Threshold=0.001
  norm : Fcn  Expr=sqrt(u(1)^2+u(2)^2+u(3)^2)
  wires:
  norm/1 -> Switch/2  "distance"
  Switch/1 -> Stop Simulation/1
  Constant1/1 -> Switch/1
  Constant2/1 -> Switch/3
  "Relative position "/1 -> norm/1

== system nonlinear_model/Stable magnet 6/stop simulation ==
  "Relative position " : Inport
  Constant1 : Constant  Value=0
  Constant2 : Constant
  Stop Simulation : Stop
  Switch : Switch  Criteria=u2 > Threshold  Threshold=0.001
  norm : Fcn  Expr=sqrt(u(1)^2+u(2)^2+u(3)^2)
  wires:
  norm/1 -> Switch/2  "distance"
  Switch/1 -> Stop Simulation/1
  Constant1/1 -> Switch/1
  Constant2/1 -> Switch/3
  "Relative position "/1 -> norm/1

== system nonlinear_model/Stable magnet 8/stop simulation ==
  "Relative position " : Inport
  Constant1 : Constant  Value=0
  Constant2 : Constant
  Stop Simulation : Stop
  Switch : Switch  Criteria=u2 > Threshold  Threshold=0.001
  norm : Fcn  Expr=sqrt(u(1)^2+u(2)^2+u(3)^2)
  wires:
  norm/1 -> Switch/2  "distance"
  Switch/1 -> Stop Simulation/1
  Constant1/1 -> Switch/1
  Constant2/1 -> Switch/3
  "Relative position "/1 -> norm/1

== system nonlinear_model/Levitujici magnet 0/Orientation computation/Angular velocity to Euler angles rates ==
  Angular velocity : Inport
  Euler angles : Inport  Port=2
  Fcn : Fcn  Expr=u(1) + ( u(2)*sin(u(4)) + u(3)*cos(u(4)) )*tan(u(5))
  Fcn1 : Fcn  Expr=u(2)*cos(u(4)) - u(3)*sin(u(4))
  Fcn2 : Fcn  Expr=( u(2)*sin(u(4)) + u(3)*cos(u(4)) )*(1/cos(u(5)))
  Mux : Mux  Inputs=2
  Mux2 : Mux  Inputs=3
  Euler angles rates : Outport
  wires:
  Fcn/1 -> Mux2/1
  Mux2/1 -> Euler angles rates/1
  Fcn2/1 -> Mux2/3
  Fcn1/1 -> Mux2/2
  Angular velocity/1 -> Mux/1
  Euler angles/1 -> Mux/2
  Mux/1 -> Fcn2/1, Fcn1/1, Fcn/1

== system nonlinear_model/Levitujici magnet 0/Orientation computation/World frame to Body frame ==
  World frame Euler angles : Inport
  World frame Vector : Inport  Port=2
  Fcn : Fcn  Expr=cos(u(5))*cos(u(6))*u(1) + cos(u(5))*sin(u(6))*u(2) - sin(u(5))*u(3)
  Fcn1 : Fcn  Expr=(-cos(u(4))*sin(u(6))+sin(u(4))*sin(u(5))*cos(u(6)))*u(1) + (cos(u(4))*cos(u(6))+sin(u(4))*sin(u(5))*sin(u(6)))*u(2) + sin(u(4))*cos(u(5))*u(3)
  Fcn2 : Fcn  Expr=(sin(u(4))*sin(u(6))+cos(u(4))*sin(u(5))*cos(u(6)))*u(1) + (-sin(u(4))*cos(u(6))+cos(u(4))*sin(u(5))*sin(u(6)))*u(2) + cos(u(4))*cos(u(5))*u(3)
  Mux : Mux  Inputs=2
  Mux1 : Mux  Inputs=2
  Mux2 : Mux  Inputs=2
  Mux3 : Mux  Inputs=3
  Body frame Vector : Outport
  wires:
  Mux/1 -> Fcn/1
  Mux1/1 -> Fcn1/1
  Mux2/1 -> Fcn2/1
  World frame Vector/1 -> Mux2/1, Mux1/1, Mux/1
  World frame Euler angles/1 -> Mux/2, Mux1/2, Mux2/2
  Mux3/1 -> Body frame Vector/1
  Fcn/1 -> Mux3/1
  Fcn1/1 -> Mux3/2
  Fcn2/1 -> Mux3/3

== system nonlinear_model/Regulators/LQR with full-state estimator/LQR ==
  state : Inport
  Demux : Demux  Outputs=2
  Gain : Gain  Gain=-K  Multiplication=Matrix(K*u)
  Saturation : Saturate  UpperLimit=max_I  LowerLimit=-max_I
  Zero-Order Hold : ZeroOrderHold  SampleTime=sample_period
  u_x : Outport
  u_y : Outport  Port=2
  wires:
  Demux/1 -> u_x/1
  Demux/2 -> u_y/1
  Gain/1 -> Saturation/1
  Saturation/1 -> Zero-Order Hold/1
  state/1 -> Gain/1
  Zero-Order Hold/1 -> Demux/1

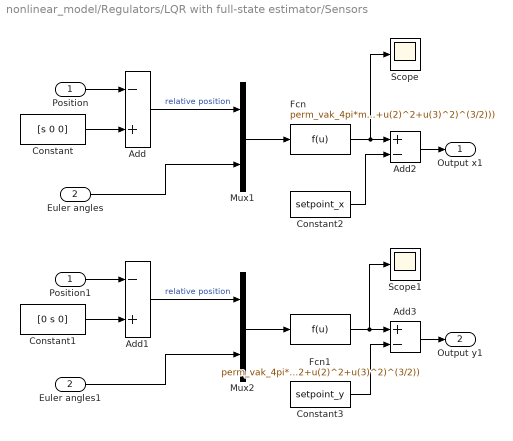
== system nonlinear_model/Regulators/LQR with full-state estimator/Sensors ==
  Position : Inport
  Euler angles : Inport  Port=2
  Add : Sum  Inputs=-+
  Add1 : Sum  Inputs=-+
  Add2 : Sum  Inputs=+-
  Add3 : Sum  Inputs=+-
  Constant : Constant  Value=[s 0 0]
  Constant1 : Constant  Value=[0 s 0]
  Constant2 : Constant  Value=setpoint_x
  Constant3 : Constant  Value=setpoint_y
  Euler angles1 : InportShadow  Port=2
  Fcn : Fcn  Expr="perm_vak_4pi*m_0 * ( (3*u(1) * ( u(1)*(sin(u(4))*sin(u(6)) + cos(u(4))*sin(u(5))*cos(u(6))) + u(2)*(-sin(u(4))*cos(u(6)) + cos(u(4))*sin(u(5))*sin(u(6))) - u(3)*(cos(u(4))*cos(u(5)))))/((u(1)^2+u(2)^2+u(3)^2)^(5/2))  -  (sin(u(4))*sin(u(6)) + cos(u(4))*sin(u(5))*cos(u(6)))/((u(1)^2+u(2)^2+u(3)^2)^(3/2)))"
  Fcn1 : Fcn  Expr="perm_vak_4pi*m_0 * ( (3*u(2) * ( u(1)*(sin(u(4))*sin(u(6))+cos(u(4))*sin(u(5))*cos(u(6))) + u(2)*(-sin(u(4))*cos(u(6))+cos(u(4))*sin(u(5))*sin(u(6))) - u(3)*(cos(u(4))*cos(u(5))) ))/(u(1)^2+u(2)^2+u(3)^2)^(5/2) -  (-sin(u(4))*cos(u(6))+cos(u(4))*sin(u(5))*sin(u(6)))/(u(1)^2+u(2)^2+u(3)^2)^(3/2))"
  Mux1 : Mux  Inputs=2
  Mux2 : Mux  Inputs=2
  Position1 : InportShadow
  Scope : Scope
  Scope1 : Scope
  Output x1 : Outport
  Output y1 : Outport  Port=2
  wires:
  Mux1/1 -> Fcn/1
  Add/1 -> Mux1/1  "relative position"
  Euler angles/1 -> Mux1/2
  Constant/1 -> Add/2
  Position/1 -> Add/1
  Mux2/1 -> Fcn1/1
  Add1/1 -> Mux2/1  "relative position"
  Euler angles1/1 -> Mux2/2
  Constant1/1 -> Add1/2
  Position1/1 -> Add1/1
  Add2/1 -> Output x1/1
  Fcn/1 -> Scope/1, Add2/1
  Constant2/1 -> Add2/2
  Fcn1/1 -> Scope1/1, Add3/1
  Add3/1 -> Output y1/1
  Constant3/1 -> Add3/2

== system nonlinear_model/Regulators/PID/PID X ==
  In1 : Inport
  Add : Sum  Inputs=3
  Discrete Derivative : simulink/Discrete/Discrete Derivative  gainval=1.0  ICPrevScaledInput=0.0  OutMin=[]  OutMax=[]  OutDataType=fixdt(1, 16)  OutScaling=2^-10  DoSatur=off
  Gain : Gain  Gain=Kp
  Gain1 : Gain  Gain=Ki
  Gain2 : Gain  Gain=Kd
  Integrator : Integrator
  Out1 : Outport
  wires:
  In1/1 -> Gain/1, Integrator/1, Discrete Derivative/1
  Integrator/1 -> Gain1/1
  Discrete Derivative/1 -> Gain2/1
  Add/1 -> Out1/1
  Gain/1 -> Add/1
  Gain1/1 -> Add/2
  Gain2/1 -> Add/3

== system nonlinear_model/Regulators/PID/PID Y ==
  In1 : Inport
  Add : Sum  Inputs=3
  Discrete Derivative : simulink/Discrete/Discrete Derivative  gainval=1.0  ICPrevScaledInput=0.0  OutMin=[]  OutMax=[]  OutDataType=fixdt(1, 16)  OutScaling=2^-10  DoSatur=off
  Gain : Gain  Gain=Kp
  Gain1 : Gain  Gain=Ki
  Gain2 : Gain  Gain=Kd
  Integrator : Integrator
  Out1 : Outport
  wires:
  Gain2/1 -> Add/3
  Gain1/1 -> Add/2
  Gain/1 -> Add/1
  Add/1 -> Out1/1
  Discrete Derivative/1 -> Gain2/1
  Integrator/1 -> Gain1/1
  In1/1 -> Discrete Derivative/1, Integrator/1, Gain/1

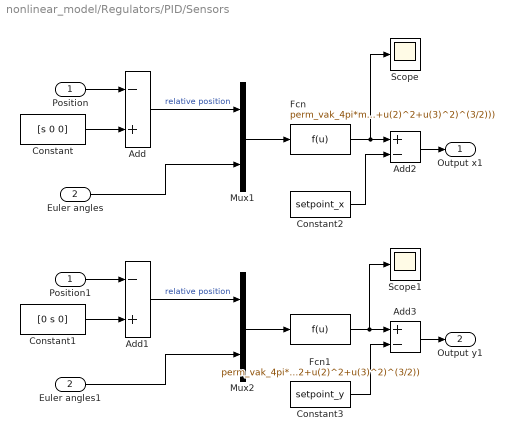
== system nonlinear_model/Regulators/PID/Sensors ==
  Position : Inport
  Euler angles : Inport  Port=2
  Add : Sum  Inputs=-+
  Add1 : Sum  Inputs=-+
  Add2 : Sum  Inputs=+-
  Add3 : Sum  Inputs=+-
  Constant : Constant  Value=[s 0 0]
  Constant1 : Constant  Value=[0 s 0]
  Constant2 : Constant  Value=setpoint_x
  Constant3 : Constant  Value=setpoint_y
  Euler angles1 : InportShadow  Port=2
  Fcn : Fcn  Expr="perm_vak_4pi*m_0 * ( (3*u(1) * ( u(1)*(sin(u(4))*sin(u(6)) + cos(u(4))*sin(u(5))*cos(u(6))) + u(2)*(-sin(u(4))*cos(u(6)) + cos(u(4))*sin(u(5))*sin(u(6))) - u(3)*(cos(u(4))*cos(u(5)))))/((u(1)^2+u(2)^2+u(3)^2)^(5/2))  -  (sin(u(4))*sin(u(6)) + cos(u(4))*sin(u(5))*cos(u(6)))/((u(1)^2+u(2)^2+u(3)^2)^(3/2)))"
  Fcn1 : Fcn  Expr="perm_vak_4pi*m_0 * ( (3*u(2) * ( u(1)*(sin(u(4))*sin(u(6))+cos(u(4))*sin(u(5))*cos(u(6))) + u(2)*(-sin(u(4))*cos(u(6))+cos(u(4))*sin(u(5))*sin(u(6))) - u(3)*(cos(u(4))*cos(u(5))) ))/(u(1)^2+u(2)^2+u(3)^2)^(5/2) -  (-sin(u(4))*cos(u(6))+cos(u(4))*sin(u(5))*sin(u(6)))/(u(1)^2+u(2)^2+u(3)^2)^(3/2))"
  Mux1 : Mux  Inputs=2
  Mux2 : Mux  Inputs=2
  Position1 : InportShadow
  Scope : Scope
  Scope1 : Scope
  Output x1 : Outport
  Output y1 : Outport  Port=2
  wires:
  Mux1/1 -> Fcn/1
  Add/1 -> Mux1/1  "relative position"
  Euler angles/1 -> Mux1/2
  Constant/1 -> Add/2
  Position/1 -> Add/1
  Mux2/1 -> Fcn1/1
  Add1/1 -> Mux2/1  "relative position"
  Euler angles1/1 -> Mux2/2
  Constant1/1 -> Add1/2
  Position1/1 -> Add1/1
  Add2/1 -> Output x1/1
  Fcn/1 -> Scope/1, Add2/1
  Constant2/1 -> Add2/2
  Fcn1/1 -> Scope1/1, Add3/1
  Add3/1 -> Output y1/1
  Constant3/1 -> Add3/2
